simulink library "constantAngleOfAttack"  (R2018a)
settings: Solver=VariableStepAuto  StartTime=0.0  StopTime=10.0  RelTol=1e-3
undefined symbols (not defined in the file): ctrl
settings Model: Creator=M.Cobb  LastModifiedBy=M.Cobb

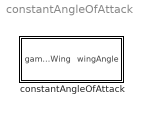
== system constantAngleOfAttack ==
  constantAngleOfAttack : Subsystem

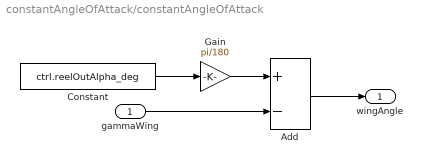
== system constantAngleOfAttack/constantAngleOfAttack ==
  gammaWing : Inport
  Add : Sum  Inputs=+-
  Constant : Constant  Value=ctrl.reelOutAlpha_deg
  Gain : Gain  Gain=pi/180
  wingAngle : Outport
  wires:
  Add/1 -> wingAngle/1
  gammaWing/1 -> Add/2
  Constant/1 -> Gain/1
  Gain/1 -> Add/1
